simulink model "VDC_testing"  (R2023b)
settings: Solver=VariableStepAuto  StartTime=0.0  StopTime=10.0  RelTol=1e-3
libraries: simulink x3
settings Model: Creator=no  LastModifiedBy=no

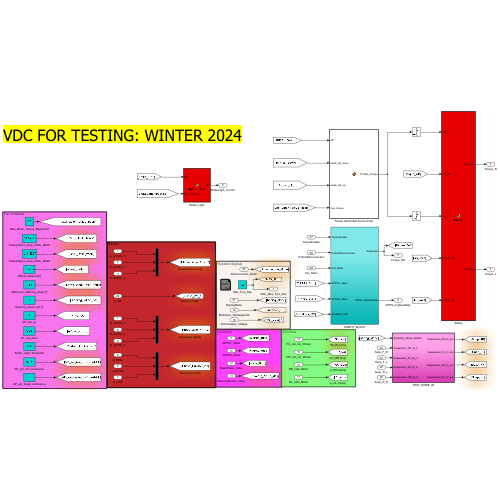
[thumbnail: Simulink's stored preview of the top-level diagram]
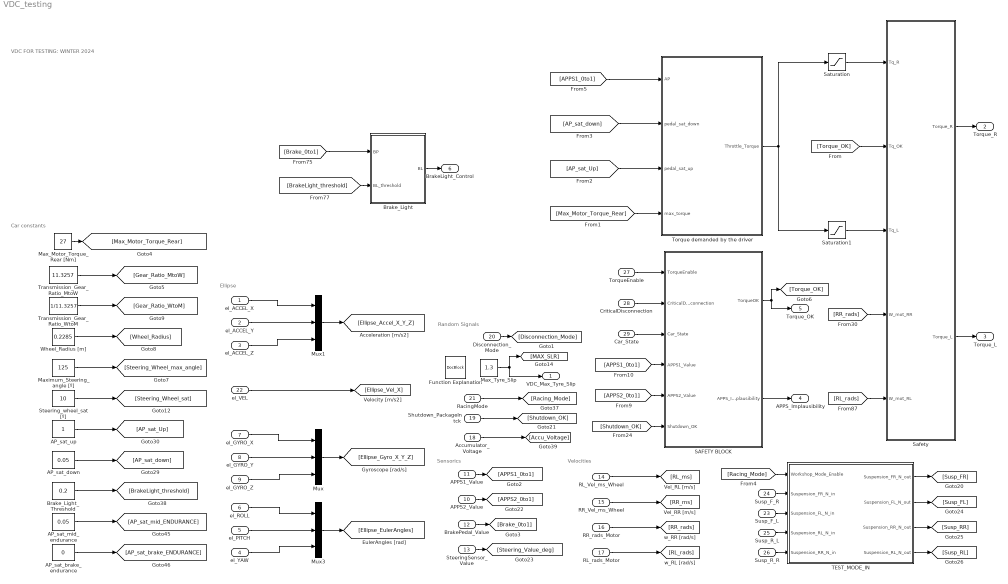
== system VDC_testing ==
  note: VDC FOR TESTING: WINTER 2024
  note: Sensorics
  note: Velocities
  note: Random Signals
  note: Car constants
  note: Ellipse
  el_ACCEL_X : Inport
  el_ACCEL_Y : Inport  Port=2
  el_ACCEL_Z : Inport  Port=3
  el_YAW : Inport  Port=4
  el_PITCH : Inport  Port=5
  el_ROLL : Inport  Port=6
  el_GYRO_X : Inport  Port=7
  el_GYRO_Y : Inport  Port=8
  el_GYRO_Z : Inport  Port=9
  APPS2_Value : Inport  Port=10
  APPS1_Value : Inport  Port=11
  BrakePedal_Value : Inport  Port=12
  SteeringSensor_Value : Inport  Port=13
  RL_Vel_ms_Wheel : Inport  Port=14
  RR_Vel_ms_Wheel : Inport  Port=15
  RR_rads_Motor : Inport  Port=16
  RL_rads_Motor : Inport  Port=17
  Accumulator_Voltage : Inport  Port=18
  Shutdown_PackageIntck : Inport  Port=19
  Disconnection_Mode : Inport  Port=20
  RacingMode : Inport  Port=21
  el_VEL : Inport  Port=22
  Susp_F_L : Inport  Port=23
  Susp_F_R : Inport  Port=24
  Susp_R_L : Inport  Port=25
  Susp_R_R : Inport  Port=26
  TorqueEnable : Inport  Port=27
  CriticalDisconnection : Inport  Port=28
  Car_State : Inport  Port=29
  AP_sat_brake_endurance : Constant  Value=0
  AP_sat_down : Constant  Value=0.05
  AP_sat_mid_endurance : Constant  Value=0.05
  AP_sat_up : Constant
  Brake_Light : MATLAB Function  TreatAsAtomicUnit=on
  Brake_Light_Threshold : Constant  Value=0.2
  Function Explanation : simulink/Model-Wide Utilities/DocBlock  DocumentType=Text
      content=|
      | Comparing the speed of the Ellipse and the speed of the Wheels, we can
      | determine the % of deviation between both (which is the slip). With
      | calculations from the Tyres & Performance Department, we know that the
      | maximum optimal slip in a STRAIGHT line is 15%. Therefore (using the Magic
      | Formula), we can determine the maximum X-Force permissible by the Wheels
      | with that % of slip (which is the constant Max_Fx_Tyre, input
      | of Rigid Axle).
      |
      | With that and the radius of the Wheels, we can calculate the maximum
      | Torque for it to stop slipping.
  Max_Motor_Torque_Rear [Nm] : Constant  Value=27
  Max_Tyre_Slip : Constant  Value=1.3
  Maximum_Steering_angle [º] : Constant  Value=125
  Mux : Mux  Inputs=3
  Mux1 : Mux  Inputs=3
  Mux3 : Mux  Inputs=3
  SAFETY BLOCK : Subsystem
  Safety : MATLAB Function  TreatAsAtomicUnit=on
  Saturation : Saturate  UpperLimit=27  LowerLimit=0
  Saturation1 : Saturate  UpperLimit=27  LowerLimit=0
  Steering_wheel_sat [º] : Constant  Value=10
  TEST_MODE_IN : Subsystem  TreatAsAtomicUnit=on
  Torque demanded by the driver : MATLAB Function  TreatAsAtomicUnit=on
  Transmission_Gear_Ratio_MtoW : Constant  Value=11.3257
  Transmission_Gear_Ratio_WtoM : Constant  Value=1/11.3257
  Wheel_Radius [m] : Constant  Value=0.2285
  VDC_Max_Tyre_Slip : Outport
  Torque_R : Outport  Port=2
  Torque_L : Outport  Port=3
  APPS_Implausibility : Outport  Port=4  VectorParamsAs1DForOutWhenUnconnected=off
  Torque_OK : Outport  Port=5  VectorParamsAs1DForOutWhenUnconnected=off
  BrakeLight_Control : Outport  Port=6  VectorParamsAs1DForOutWhenUnconnected=off
  wires:
  APPS2_Value/1 -> [APPS2_0to1]
  Maximum_Steering_angle [º]/1 -> [Steering_Wheel_max_angle]
  Disconnection_Mode/1 -> [Disconnection_Mode]
  Wheel_Radius [m]/1 -> [Wheel_Radius]
  el_ROLL/1 -> Mux3/1
  el_VEL/1 -> [Ellipse_Vel_X]
  RR_rads_Motor/1 -> [RR_rads]
  AP_sat_mid_endurance/1 -> [AP_sat_mid_ENDURANCE]
  Transmission_Gear_Ratio_WtoM/1 -> [Gear_Ratio_WtoM]
  Transmission_Gear_Ratio_MtoW/1 -> [Gear_Ratio_MtoW]
  el_PITCH/1 -> Mux3/2
  Brake_Light_Threshold/1 -> [BrakeLight_threshold]
  SteeringSensor_Value/1 -> [Steering_Value_deg]
  RL_rads_Motor/1 -> [RL_rads]
  RacingMode/1 -> [Racing_Mode]
  Max_Tyre_Slip/1 -> [MAX_SLR], VDC_Max_Tyre_Slip/1
  AP_sat_down/1 -> [AP_sat_down]
  BrakePedal_Value/1 -> [Brake_0to1]
  RR_Vel_ms_Wheel/1 -> [RR_ms]
  Max_Motor_Torque_Rear [Nm]/1 -> [Max_Motor_Torque_Rear]
  APPS1_Value/1 -> [APPS1_0to1]
  AP_sat_brake_endurance/1 -> [AP_sat_brake_ENDURANCE]
  Accumulator_Voltage/1 -> [Accu_Voltage]
  el_YAW/1 -> Mux3/3
  el_GYRO_Z/1 -> Mux/3
  Mux1/1 -> [Ellipse_Accel_X_Y_Z]
  el_GYRO_Y/1 -> Mux/2
  AP_sat_up/1 -> [AP_sat_Up]
  Mux3/1 -> [Ellipse_EulerAngles]
  RL_Vel_ms_Wheel/1 -> [RL_ms]
  el_GYRO_X/1 -> Mux/1
  el_ACCEL_Z/1 -> Mux1/3
  Mux/1 -> [Ellipse_Gyro_X_Y_Z]
  el_ACCEL_Y/1 -> Mux1/2
  el_ACCEL_X/1 -> Mux1/1
  Steering_wheel_sat [º]/1 -> [Steering_Wheel_sat]
  Shutdown_PackageIntck/1 -> [Shutdown_OK]
  [RL_rads] -> Safety/5(W_mot_RL)
  Saturation1/1 -> Safety/3(Tq_L)
  Safety/1(Torque_R) -> Torque_R/1
  Safety/2(Torque_L) -> Torque_L/1
  [RR_rads] -> Safety/4(W_mot_RR)
  Saturation/1 -> Safety/1(Tq_R)
  [Shutdown_OK] -> SAFETY BLOCK/6(Shutdown_OK)
  [APPS2_0to1] -> SAFETY BLOCK/5(APPS2_Value)
  [APPS1_0to1] -> SAFETY BLOCK/4(APPS1_Value)
  CriticalDisconnection/1 -> SAFETY BLOCK/2(CriticalDisconnection)
  TEST_MODE_IN/1(Suspension_FR_N_out) -> [Susp_FR]
  TorqueEnable/1 -> SAFETY BLOCK/1(TorqueEnable)
  Car_State/1 -> SAFETY BLOCK/3(Car_State)
  TEST_MODE_IN/2(Suspension_FL_N_out) -> [Susp_FL]
  SAFETY BLOCK/2(APPS_Implausibility) -> APPS_Implausibility/1
  TEST_MODE_IN/4(Suspension_RL_N_out) -> [Susp_RL]
  Susp_F_L/1 -> TEST_MODE_IN/3(Suspension_FL_N_in)
  Susp_R_R/1 -> TEST_MODE_IN/5(Suspension_RR_N_in)
  Susp_F_R/1 -> TEST_MODE_IN/2(Suspension_FR_N_in)
  TEST_MODE_IN/3(Suspension_RR_N_out) -> [Susp_RR]
  [BrakeLight_threshold] -> Brake_Light/2(BL_threshold)
  Susp_R_L/1 -> TEST_MODE_IN/4(Suspension_RL_N_in)
  [Brake_0to1] -> Brake_Light/1(BP)
  [Racing_Mode] -> TEST_MODE_IN/1(Workshop_Mode_Enable)
  SAFETY BLOCK/1(TorqueOK) -> Torque_OK/1, [Torque_OK]
  Brake_Light/1(BL) -> BrakeLight_Control/1
  [Torque_OK] -> Safety/2(Tq_OK)
  Torque demanded by the driver/1(Throttle_Torque) -> Saturation/1, Saturation1/1
  [Max_Motor_Torque_Rear] -> Torque demanded by the driver/4(max_torque)
  [AP_sat_down] -> Torque demanded by the driver/2(pedal_sat_down)
  [AP_sat_Up] -> Torque demanded by the driver/3(pedal_sat_up)
  [APPS1_0to1] -> Torque demanded by the driver/1(AP)

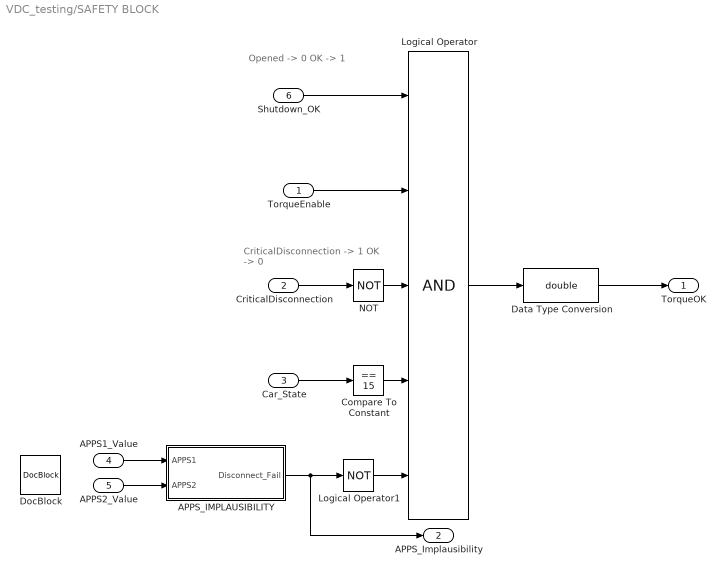
== system VDC_testing/SAFETY BLOCK ==
  note: CriticalDisconnection -> 1
      | OK -> 0
  note: Opened -> 0
      | OK -> 1
  TorqueEnable : Inport
  CriticalDisconnection : Inport  Port=2
  Car_State : Inport  Port=3
  APPS1_Value : Inport  Port=4
  APPS2_Value : Inport  Port=5
  Shutdown_OK : Inport  Port=6
  APPS_IMPLAUSIBILITY : Subsystem
  Compare To Constant : simulink/Logic and Bit Operations/Compare To Constant  relop===  const=15  OutDataTypeStr=boolean
  Data Type Conversion : DataTypeConversion  OutDataTypeStr=double  SaturateOnIntegerOverflow=off  RndMeth=Floor
  DocBlock : simulink/Model-Wide Utilities/DocBlock  DocumentType=Text
      content=|
      | Formula Student Rules 2024 -> T11.8.8
      |     If an implausibility occurs between the values of the APPSs and
      |     persists for more than 100 ms:
      |     • [EV ONLY] The power to the motor(s) must be immediately shut down
      |     completely. It is not necessary to completely deactivate the TS, the
      |     motor controller(s) shutting down the power to the motor(s) is
      |     sufficient.
      |
      | The 'Number_of_Periods' constant, if there's an Implausability, outputs the error X
      | periods (100ms) after the Implausibility happened (25ms * X = 100ms).
  Logical Operator : Logic  Inputs=5  OutDataTypeStr=boolean
  Logical Operator1 : Logic  Operator=NOT  IconShape=distinctive  AllPortsSameDT=off  OutDataTypeStr=boolean
  NOT : Logic  Operator=NOT  IconShape=distinctive  AllPortsSameDT=off  OutDataTypeStr=boolean
  TorqueOK : Outport  VectorParamsAs1DForOutWhenUnconnected=off
  APPS_Implausibility : Outport  Port=2  VectorParamsAs1DForOutWhenUnconnected=off
  wires:
  Logical Operator/1 -> Data Type Conversion/1
  Car_State/1 -> Compare To Constant/1
  NOT/1 -> Logical Operator/3
  CriticalDisconnection/1 -> NOT/1
  TorqueEnable/1 -> Logical Operator/2
  APPS2_Value/1 -> APPS_IMPLAUSIBILITY/2(APPS2)
  APPS1_Value/1 -> APPS_IMPLAUSIBILITY/1(APPS1)
  APPS_IMPLAUSIBILITY/1(Disconnect_Fail) -> APPS_Implausibility/1, Logical Operator1/1
  Compare To Constant/1 -> Logical Operator/4
  Shutdown_OK/1 -> Logical Operator/1
  Logical Operator1/1 -> Logical Operator/5
  Data Type Conversion/1 -> TorqueOK/1

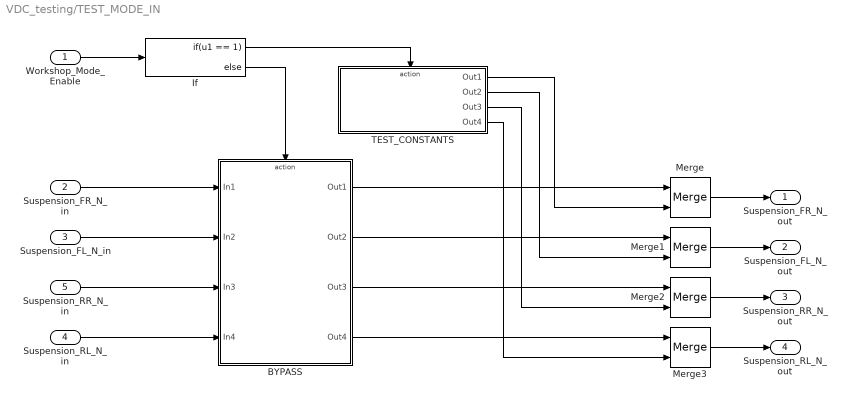
== system VDC_testing/TEST_MODE_IN ==
  Workshop_Mode_Enable : Inport
  Suspension_FR_N_in : Inport  Port=2
  Suspension_FL_N_in : Inport  Port=3
  Suspension_RL_N_in : Inport  Port=4
  Suspension_RR_N_in : Inport  Port=5
  BYPASS : Subsystem  TreatAsAtomicUnit=on
  If : If  IfExpression=u1 == 1
  Merge{,1..3} (4 alike) : Merge
  TEST_CONSTANTS : Subsystem  TreatAsAtomicUnit=on
  Suspension_FR_N_out : Outport  VectorParamsAs1DForOutWhenUnconnected=off
  Suspension_FL_N_out : Outport  Port=2  VectorParamsAs1DForOutWhenUnconnected=off
  Suspension_RR_N_out : Outport  Port=3  VectorParamsAs1DForOutWhenUnconnected=off
  Suspension_RL_N_out : Outport  Port=4  VectorParamsAs1DForOutWhenUnconnected=off
  wires:
  Suspension_FR_N_in/1 -> BYPASS/1(In1)
  Suspension_FL_N_in/1 -> BYPASS/2(In2)
  Suspension_RR_N_in/1 -> BYPASS/3(In3)
  Suspension_RL_N_in/1 -> BYPASS/4(In4)
  Merge/1 -> Suspension_FR_N_out/1
  Merge1/1 -> Suspension_FL_N_out/1
  Merge2/1 -> Suspension_RR_N_out/1
  Merge3/1 -> Suspension_RL_N_out/1
  BYPASS/1(Out1) -> Merge/1
  BYPASS/2(Out2) -> Merge1/1
  BYPASS/3(Out3) -> Merge2/1
  BYPASS/4(Out4) -> Merge3/1
  Workshop_Mode_Enable/1 -> If/1
  If/2 -> BYPASS/Action
  If/1 -> TEST_CONSTANTS/Action
  TEST_CONSTANTS/4(Out4) -> Merge3/2
  TEST_CONSTANTS/3(Out3) -> Merge2/2
  TEST_CONSTANTS/2(Out2) -> Merge1/2
  TEST_CONSTANTS/1(Out1) -> Merge/2

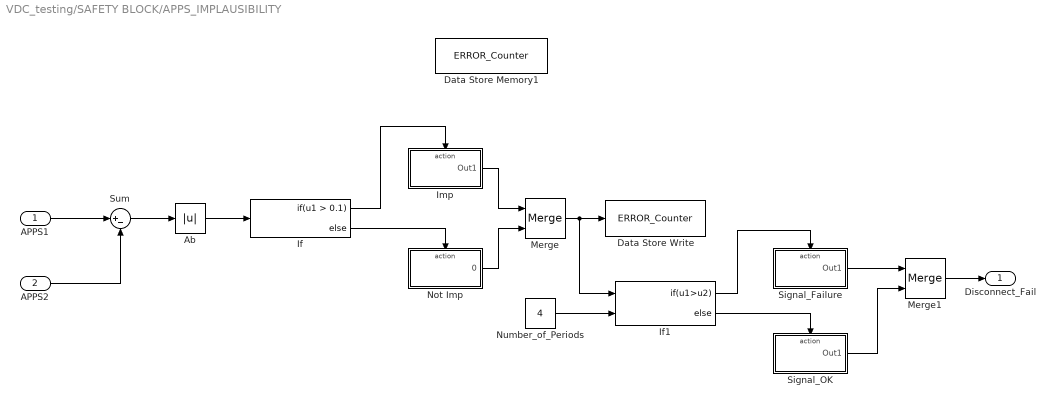
== system VDC_testing/SAFETY BLOCK/APPS_IMPLAUSIBILITY ==
  APPS1 : Inport
  APPS2 : Inport  Port=2
  Ab : Abs  SaturateOnIntegerOverflow=off
  Data Store Memory1 : DataStoreMemory  DataStoreName=ERROR_Counter  ReadBeforeWriteMsg=warning  WriteAfterWriteMsg=warning  WriteAfterReadMsg=warning  ShowAdditionalParam=off
  Data Store Write : DataStoreWrite  DataStoreName=ERROR_Counter  IndexOptions=Index vector (dialog)  Indices=1  OutputSizes=1
  If : If  IfExpression=u1 > 0.1
  If1 : If  NumInputs=2  IfExpression=u1>u2
  Imp : Subsystem  TreatAsAtomicUnit=on
  Merge : Merge
  Merge1 : Merge
  Not Imp : Subsystem  TreatAsAtomicUnit=on
  Number_of_Periods : Constant  Value=4
  Signal_Failure : Subsystem  TreatAsAtomicUnit=on
  Signal_OK : Subsystem  TreatAsAtomicUnit=on
  Sum : Sum  Inputs=|+-
  Disconnect_Fail : Outport  VectorParamsAs1DForOutWhenUnconnected=off
  wires:
  Number_of_Periods/1 -> If1/2
  Imp/1(Out1) -> Merge/1
  Signal_Failure/1(Out1) -> Merge1/1
  Signal_OK/1(Out1) -> Merge1/2
  Merge1/1 -> Disconnect_Fail/1
  APPS1/1 -> Sum/1
  If/1 -> Imp/Action
  If1/2 -> Signal_OK/Action
  Merge/1 -> Data Store Write/1, If1/1
  If1/1 -> Signal_Failure/Action
  APPS2/1 -> Sum/2
  Ab/1 -> If/1
  If/2 -> Not Imp/Action
  Sum/1 -> Ab/1
  Not Imp/1(0) -> Merge/2

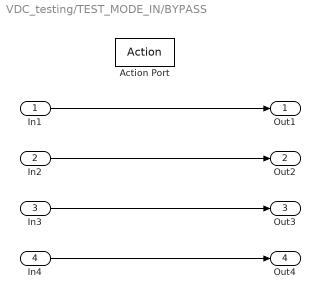
== system VDC_testing/TEST_MODE_IN/BYPASS ==
  In1 : Inport
  In2 : Inport  Port=2
  In3 : Inport  Port=3
  In4 : Inport  Port=4
  Action Port : ActionPort
  Out1 : Outport  VectorParamsAs1DForOutWhenUnconnected=off
  Out2 : Outport  Port=2  VectorParamsAs1DForOutWhenUnconnected=off
  Out3 : Outport  Port=3  VectorParamsAs1DForOutWhenUnconnected=off
  Out4 : Outport  Port=4  VectorParamsAs1DForOutWhenUnconnected=off
  wires:
  In1/1 -> Out1/1
  In2/1 -> Out2/1
  In3/1 -> Out3/1
  In4/1 -> Out4/1

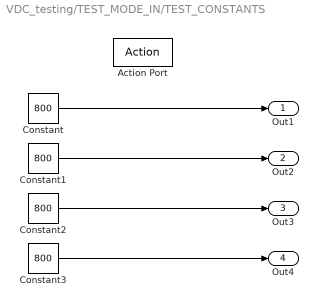
== system VDC_testing/TEST_MODE_IN/TEST_CONSTANTS ==
  Action Port : ActionPort
  Constant{,1..3} (4 alike) : Constant  Value=800
  Out1 : Outport  VectorParamsAs1DForOutWhenUnconnected=off
  Out2 : Outport  Port=2  VectorParamsAs1DForOutWhenUnconnected=off
  Out3 : Outport  Port=3  VectorParamsAs1DForOutWhenUnconnected=off
  Out4 : Outport  Port=4  VectorParamsAs1DForOutWhenUnconnected=off
  wires:
  Constant/1 -> Out1/1
  Constant1/1 -> Out2/1
  Constant2/1 -> Out3/1
  Constant3/1 -> Out4/1

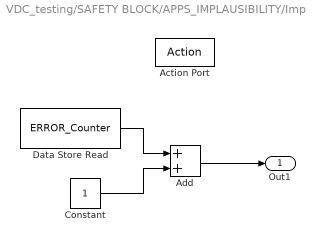
== system VDC_testing/SAFETY BLOCK/APPS_IMPLAUSIBILITY/Imp ==
  Action Port : ActionPort
  Add : Sum
  Constant : Constant  OutDataTypeStr=boolean
  Data Store Read : DataStoreRead  DataStoreName=ERROR_Counter  IndexOptions=Index vector (dialog)  Indices=1  OutputSizes=1
  Out1 : Outport  VectorParamsAs1DForOutWhenUnconnected=off
  wires:
  Data Store Read/1 -> Add/1
  Constant/1 -> Add/2
  Add/1 -> Out1/1

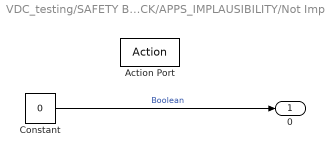
== system VDC_testing/SAFETY BLOCK/APPS_IMPLAUSIBILITY/Not Imp ==
  Action Port : ActionPort
  Constant : Constant  Value=0  OutDataTypeStr=double
  0 : Outport  VectorParamsAs1DForOutWhenUnconnected=off
  wires:
  Constant/1 -> 0/1  "Boolean"

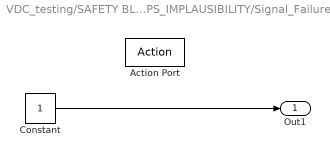
== system VDC_testing/SAFETY BLOCK/APPS_IMPLAUSIBILITY/Signal_Failure ==
  Action Port : ActionPort
  Constant : Constant
  Out1 : Outport  VectorParamsAs1DForOutWhenUnconnected=off
  wires:
  Constant/1 -> Out1/1

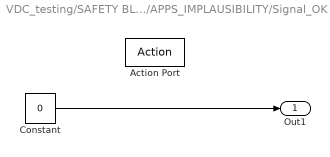
== system VDC_testing/SAFETY BLOCK/APPS_IMPLAUSIBILITY/Signal_OK ==
  Action Port : ActionPort
  Constant : Constant  Value=0
  Out1 : Outport  VectorParamsAs1DForOutWhenUnconnected=off
  wires:
  Constant/1 -> Out1/1

== matlab function VDC_testing/Brake_Light ==
  data: BP input; BL output; BL_threshold input
function BL = Brake_Light(BP, BL_threshold)
    if (BP > BL_threshold)
        BL = 1;
        return;
    else
        BL = 0;
        return;
    end
end

== matlab function VDC_testing/Safety ==
  data: Tq_R input; Tq_OK input; Tq_L input; Torque_R output; Torque_L output; W_mot_RR input; W_mot_RL input
function [Torque_R,Torque_L]  = Safety(Tq_R, Tq_OK, Tq_L, W_mot_RR, W_mot_RL)
    if Tq_OK == 1 && max(W_mot_RR, W_mot_RL < 1250
        Torque_R = Tq_R;
        Torque_L = Tq_L;
        return;
    else
        Torque_R = 0;
        Torque_L = 0;
        return;
    end
end

== matlab function VDC_testing/Torque demanded by the driver ==
  data: Throttle_Torque output; AP input; pedal_sat_down input; pedal_sat_up input; max_torque input
function Throttle_Torque  = TT(AP, pedal_sat_down, pedal_sat_up, max_torque)
    if AP <= pedal_sat_down %establish the lower deadzone for the throttle pedal
        Throttle_Response = 0;

    elseif AP >= pedal_sat_up %establish the higher deadzone for the throttle pedal
        Throttle_Response = 1;

    else
        Throttle_Response = ((AP - pedal_sat_down) / (pedal_sat_up - pedal_sat_down)); %evaluate for given input
    end
    Throttle_Torque = Throttle_Response * max_torque; % set torque to max output times pedal factor
end
